simulink model "step6_ref"  (Simulink 10.2)
settings: Solver=FixedStepAuto  StartTime=0.0  StopTime=3  FixedStep=T_step  RelTol=1e-3
values from neighbouring files (symbols this model uses):
  gama0 = Rparams4dyn(3)    [PRBDM_3R_Dynamic_Matrices_Lagrange.m]    (also in PRBDM_3R_Dynamics.m = in4dyn(12); PRBDM_3R_Dynamics00.m = in4dyn(12); PRBDM_3R_DynamicsPID.m = in4dyn(12); PRBDM_3R_parameters.m = 0.1)
  gama1 = x(7)    [Jacobi_T.m]    (also in PRBDM_3R_Dynamic_Matrices_Lagrange.m = Rparams4dyn(4); PRBDM_3R_Dynamics.m = in4dyn(13); PRBDM_3R_Dynamics00.m = in4dyn(13); PRBDM_3R_DynamicsPID.m = in4dyn(13))
  gama2 = x(8)    [Jacobi_T.m]    (also in PRBDM_3R_Dynamic_Matrices_Lagrange.m = Rparams4dyn(5); PRBDM_3R_Dynamics.m = in4dyn(14); PRBDM_3R_Dynamics00.m = in4dyn(14); PRBDM_3R_DynamicsPID.m = in4dyn(14))
  gama3 = x(9)    [Jacobi_T.m]    (also in PRBDM_3R_Dynamic_Matrices_Lagrange.m = Rparams4dyn(6); PRBDM_3R_Dynamics.m = in4dyn(15); PRBDM_3R_Dynamics00.m = in4dyn(15); PRBDM_3R_DynamicsPID.m = in4dyn(15))
  I = Rparams4dyn(10)    [PRBDM_3R_Dynamic_Matrices_Lagrange.m]    (also in PRBDM_3R_Dynamics.m = in4dyn(19); PRBDM_3R_Dynamics00.m = in4dyn(19); PRBDM_3R_DynamicsPID.m = in4dyn(19); PRBDM_3R_parameters.m = 1.8e-11)
  k1 = Rparams4dyn(7)    [PRBDM_3R_Dynamic_Matrices_Lagrange.m]    (also in PRBDM_3R_Dynamics.m = in4dyn(16); PRBDM_3R_Dynamics00.m = in4dyn(16); PRBDM_3R_DynamicsPID.m = in4dyn(16); PRBDM_3R_parameters.m = 0.290628)
  k2 = Rparams4dyn(8)    [PRBDM_3R_Dynamic_Matrices_Lagrange.m]    (also in PRBDM_3R_Dynamics.m = in4dyn(17); PRBDM_3R_Dynamics00.m = in4dyn(17); PRBDM_3R_DynamicsPID.m = in4dyn(17); PRBDM_3R_parameters.m = 0.247572)
  k3 = Rparams4dyn(9)    [PRBDM_3R_Dynamic_Matrices_Lagrange.m]    (also in PRBDM_3R_Dynamics.m = in4dyn(18); PRBDM_3R_Dynamics00.m = in4dyn(18); PRBDM_3R_DynamicsPID.m = in4dyn(18); PRBDM_3R_parameters.m = 0.213624)
  L = Rparams4dyn(2)    [PRBDM_3R_Dynamic_Matrices_Lagrange.m]    (also in PRBDM_3R_Dynamics.m = in4dyn(11); PRBDM_3R_Dynamics00.m = in4dyn(11); PRBDM_3R_DynamicsPID.m = in4dyn(11); PRBDM_3R_parameters.m = 0.3)
  m = Rparams4dyn(1)    [PRBDM_3R_Dynamic_Matrices_Lagrange.m]    (also in PRBDM_3R_Dynamics.m = in4dyn(10); PRBDM_3R_Dynamics00.m = in4dyn(10); PRBDM_3R_DynamicsPID.m = in4dyn(10); PRBDM_3R_parameters.m = 1)
  W = x(22)    [PRBDM_3R_CTC.m]    (also in PRBDM_3R_Dynamic_Matrices_NewtonEular.m = robot_params(7); PRBDM_3R_Dynamics.m = in4dyn(20); PRBDM_3R_Dynamics00.m = in4dyn(20); PRBDM_3R_DynamicsPID.m = in4dyn(20))
libraries: pid_lib x1
settings Model: Creator=Master  LastModifiedBy=Master
settings DataIOCC: SaveFormat=Dataset  SignalLoggingSaveFormat=Dataset  ReturnWorkspaceOutputs=on
settings OptimizationCC: LifeSpan=auto
settings DebuggingCC: UnderspecifiedInitializationDetection=Simplified  MergeDetectMultiDrivingBlocksExec=error  FcnCallInpInsideContextMsg=error  SFUnexpectedBacktrackingDiag=error  SFNoUnconditionalDefaultTransitionDiag=error  SFExecutionAtInitializationDiag=warning  ArithmeticOperatorsInVariantConditions=error
settings HardwareCC: ProdBitPerPointer=64  ProdBitPerSizeT=64  ProdBitPerPtrDiffT=64  ProdLargestAtomicFloat=Float  ProdIntDivRoundTo=Zero  ProdEndianess=LittleEndian  ProdWordSize=64  ProdHWDeviceType=Intel->x86-64 (Windows64)
settings ModelReferenceCC: PropagateSignalLabelsOutOfModel=on
settings SFSimCC: SimUseLocalCustomCode=on  CustomCodeUndefinedFunction=FilterOut
settings RTWCC: RTWUseLocalCustomCode=on
settings CodeAppCC: StateflowObjectComments=off
settings GRTTargetCC: TargetLangStandard=C99 (ISO)  CombineOutputUpdateFcns=on  GRTInterface=off
settings ConfigComp: CovMetricSettings=dwe  CovSaveCumulativeToWorkspaceVar=off  CovSaveSingleToWorkspaceVar=off  CovExternalEMLEnable=on

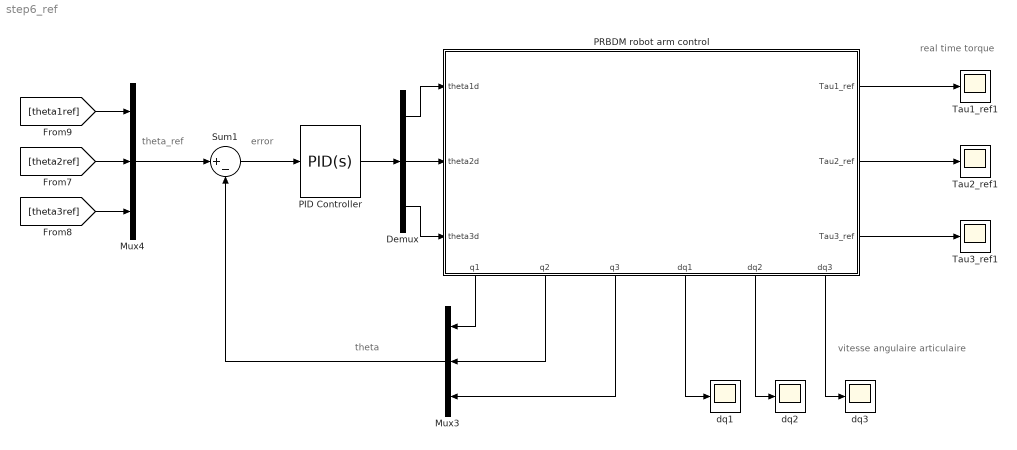
== system step6_ref ==
  note: vitesse angulaire articulaire
  note: real time torque
  note: theta
  note: theta_ref
  note: error
  " dq1" : Scope
  Demux : Demux  Outputs=3
  Mux3 : Mux  Inputs=3
  Mux4 : Mux  Inputs=3
  PID Controller : pid_lib/PID Controller  Controller=PID  Form=Parallel  TimeDomain=Continuous-time  UseExternalTs=off  SampleTime=-1  IntegratorMethod=Forward Euler  FilterMethod=Forward Euler  ControllerParametersSource=internal  P=1  I=1  D=0  UseFilter=on  N=100  TunerSelectOption=Transfer Function Based (PID Tuner App)  InitialConditionSource=internal  InitialConditionForIntegrator=0  InitialConditionForFilter=0  DifferentiatorICPrevScaledInput=0  ExternalReset=none  TrackingMode=off  Kt=1  LimitOutput=off  SatLimitsSource=internal  UpperSaturationLimit=inf  LowerSaturationLimit=-inf  LinearizeAsGain=on  AntiWindupMode=none  Kb=1  POutMin=[]  POutMax=[]  IOutMin=[]  IOutMax=[]  DOutMin=[]  DOutMax=[]  NOutMin=[]  NOutMax=[]  SumOutMin=[]  SumOutMax=[]  SaturationOutMin=[]  SaturationOutMax=[]  PParamMin=[]  PParamMax=[]  IParamMin=[]  IParamMax=[]  DParamMin=[]  DParamMax=[]  NParamMin=[]  NParamMax=[]  KbParamMin=[]  KbParamMax=[]  KtParamMin=[]  KtParamMax=[]  KbOutMin=[]  KbOutMax=[]  KtOutMin=[]  KtOutMax=[]  IntegratorOutMin=[]  IntegratorOutMax=[]  FilterOutMin=[]  FilterOutMax=[]  SumI1OutMin=[]  SumI1OutMax=[]  SumI2OutMin=[]  SumI2OutMax=[]  SumI3OutMin=[]  SumI3OutMax=[]  SumI4OutMin=[]  SumI4OutMax=[]  SumDOutMin=[]  SumDOutMax=[]  DifferentiatorOutMin=[]  DifferentiatorOutMax=[]  FilterDiffOutCoefMin=[]  FilterDiffOutCoefMax=[]  ReciprocalOutMin=[]  ReciprocalOutMax=[]  SumDenOutMin=[]  SumDenOutMax=[]  SumNumOutMin=[]  SumNumOutMax=[]  DivideOutMin=[]  DivideOutMax=[]  UdiffTsProdOutMin=[]  UdiffTsProdOutMax=[]  NTsProdOutMin=[]  NTsProdOutMax=[]  UintegralTsProdOutMin=[]  UintegralTsProdOutMax=[]  UngainTsProdOutMin=[]  UngainTsProdOutMax=[]  IntegratorContinuousStateAttributes=''  IntegratorStateMustResolveToSignalObject=off  IntegratorRTWStateStorageClass=Auto  FilterContinuousStateAttributes=''  FilterStateMustResolveToSignalObject=off  FilterRTWStateStorageClass=Auto  ParallelPVariant=InternalParameters  IdealPVariant=Disabled  IVariant=InternalParameters  DVariant=InternalParameters  IntegratorVariant=Continuous  SatVariant=Disabled  AWVariant=Passthrough  PCopyVariant=Disabled  TRVariant=Disabled  FdbkBlocksVariant=Forward  IdealPFdbkVariant=Disabled  SatFdbkVariant=Disabled  DerivativeFilterVariant=ContFilter  NVariant=InternalParameters  NCopyVariant=Disabled  FilterICVariant=InternalICsFilter  IntegratorICVariant=InternalICs  ExternalResetVariant=Disabled  TRSumVariant=Passthrough  SumFdbkVariant=Disabled  SumVariant=Sum_PID  TsampFilterVariant=InternalTs  TsampNgainVariant=Passthrough  TsampIntegralVariant=Passthrough  ExternalSaturationOutDataTypeStr=Inherit: Same as second input
  PRBDM robot arm control : Subsystem
      settings: PortSchema="{\"entries\":[{\"content\":{\"sides\":[{\"content\":{\"connectorIds\":[\"In1\",\"In2\",\"In3\"]},\"type\":\"ConnectorPlacement.EquallySpacedRectSide\",\"uuid\":\"1e89617d-77c4-4021-ad02-b23032c49c13\"},{\"content\":{\"connectorIds\":[\"Out1\",\"Out2\",\"Out3\"],\"side\":\"RIGHT\"},\"type\":\"ConnectorPlacement.EquallySpacedRectSide\",\"uuid\":\"af1c966f-61d8-4dd1-b14e-ca4c94ca536d\"},{\"content\":{\"connectorIds\":[],\"side\":\"TOP\"},\"type\":\"ConnectorPlacement.EquallySpacedRectSide\",\"uuid\":\"dae36e8b-a61f-4fb2-b828-973ce72430cd\"},{\"content\":{\"connectorIds\":[\"Out4\",\"Out5\",\"Out6\",\"Out7\",\"Out8\",\"Out9\"],\"side\":\"BOTTOM\"},\"type\":\"ConnectorPlacement.EquallySpacedRectSide\",\"uuid\":\"432115d0-4cd6-420b-9ede-52c2ebd6cc12\"},{\"content\":{\"connectorIds\":[],\"side\":\"HIDDEN\"},\"type\":\"ConnectorPlacement.EquallySpacedRectSide\",\"uuid\":\"bc2aa4ed-b8ff-4e0b-a675-9c9f1376083d\"}]},\"type\":\"ConnectorPlacement.EquallySpacedConnector\",\"uuid\":\"b45c6bc8-8dc8-4362-beb6-c8f75c6afe37\"}],\"packageUris\":[\"http://schema.mathworks.com/mf0/Connector/R2020b\"],\"version\":\"1.0\"}"
      mask Display: image(imread('RRR.png'))
  Sum1 : Sum  Inputs=|+-
  Tau1_ref1 : Scope
  Tau2_ref1 : Scope
  Tau3_ref1 : Scope
  dq2 : Scope
  dq3 : Scope
  wires:
  PRBDM robot arm control/4(q1) -> Mux3/1
  [theta2ref] -> Mux4/2
  [theta3ref] -> Mux4/3
  [theta1ref] -> Mux4/1
  Mux4/1 -> Sum1/1
  Mux3/1 -> Sum1/2
  Sum1/1 -> PID Controller/1
  PID Controller/1 -> Demux/1
  Demux/2 -> PRBDM robot arm control/2(theta2d)
  Demux/1 -> PRBDM robot arm control/1(theta1d)
  Demux/3 -> PRBDM robot arm control/3(theta3d)
  PRBDM robot arm control/5(q2) -> Mux3/2
  PRBDM robot arm control/6(q3) -> Mux3/3
  PRBDM robot arm control/7(dq1) -> " dq1"/1
  PRBDM robot arm control/8(dq2) -> dq2/1
  PRBDM robot arm control/9(dq3) -> dq3/1
  PRBDM robot arm control/2(Tau2_ref) -> Tau2_ref1/1
  PRBDM robot arm control/1(Tau1_ref) -> Tau1_ref1/1
  PRBDM robot arm control/3(Tau3_ref) -> Tau3_ref1/1

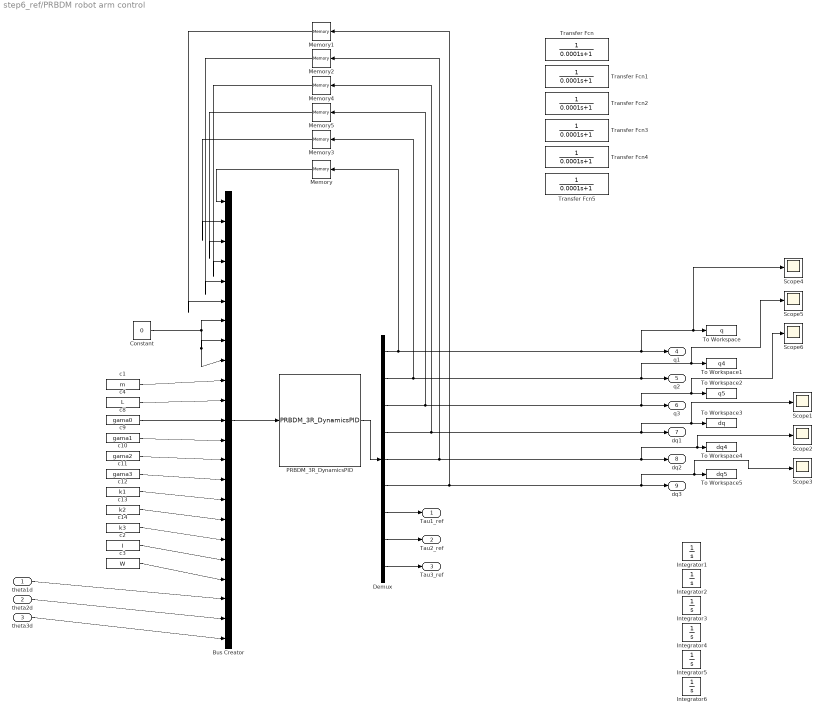
== system step6_ref/PRBDM robot arm control ==
  theta1d : Inport
  theta2d : Inport  Port=2
  theta3d : Inport  Port=3
  Bus Creator : BusCreator  Inputs=23
  Constant : Constant  Value=0
  Demux : Demux  Outputs=9
  Integrator{1..6} (6 alike) : Integrator  UpperSaturationLimit=1e6  LowerSaturationLimit=-1e6
  Memory{,1..5} (6 alike) : Memory
  PRBDM_3R_DynamicsPID : MATLABFcn  MATLABFcn=PRBDM_3R_DynamicsPID  OutputDimensions=9
  Scope{1..6} (6 alike) : Scope
  To Workspace : ToWorkspace  VariableName=q  SampleTime=-1
  To Workspace1 : ToWorkspace  VariableName=q4  SampleTime=-1
  To Workspace2 : ToWorkspace  VariableName=q5  SampleTime=-1
  To Workspace3 : ToWorkspace  VariableName=dq  SampleTime=-1
  To Workspace4 : ToWorkspace  VariableName=dq4  SampleTime=-1
  To Workspace5 : ToWorkspace  VariableName=dq5  SampleTime=-1
  Transfer Fcn{,1..5} (6 alike) : TransferFcn  Denominator=[0.0001 1]
  c1 : Constant  Value=m
  c10 : Constant  Value=gama2
  c11 : Constant  Value=gama3
  c12 : Constant  Value=k1
  c13 : Constant  Value=k2
  c14 : Constant  Value=k3
  c2 : Constant  Value=I
  c3 : Constant  Value=W
  c4 : Constant  Value=L
  c8 : Constant  Value=gama0
  c9 : Constant  Value=gama1
  Tau1_ref : Outport
  Tau2_ref : Outport  Port=2
  Tau3_ref : Outport  Port=3
  q1 : Outport  Port=4
  q2 : Outport  Port=5
  q3 : Outport  Port=6
  dq1 : Outport  Port=7
  dq2 : Outport  Port=8
  dq3 : Outport  Port=9
  wires:
  theta3d/1 -> Bus Creator/23
  theta2d/1 -> Bus Creator/22
  c11/1 -> Bus Creator/15
  c3/1 -> Bus Creator/20
  c14/1 -> Bus Creator/18
  c2/1 -> Bus Creator/19
  c1/1 -> Bus Creator/10
  c8/1 -> Bus Creator/12
  Bus Creator/1 -> PRBDM_3R_DynamicsPID/1
  PRBDM_3R_DynamicsPID/1 -> Demux/1
  c4/1 -> Bus Creator/11
  c10/1 -> Bus Creator/14
  c9/1 -> Bus Creator/13
  c13/1 -> Bus Creator/17
  c12/1 -> Bus Creator/16
  theta1d/1 -> Bus Creator/21
  Demux/1 -> Memory/1, q1/1, Scope4/1, To Workspace/1
  Demux/2 -> Memory3/1, q2/1, Scope5/1, To Workspace1/1
  Demux/3 -> Memory5/1, q3/1, Scope6/1, To Workspace2/1
  Demux/4 -> Memory4/1, dq1/1, Scope1/1, To Workspace3/1
  Demux/5 -> Memory2/1, dq2/1, Scope2/1, To Workspace4/1
  Demux/6 -> Memory1/1, dq3/1, Scope3/1, To Workspace5/1
  Memory/1 -> Bus Creator/1
  Memory3/1 -> Bus Creator/2
  Memory5/1 -> Bus Creator/3
  Memory4/1 -> Bus Creator/4
  Memory2/1 -> Bus Creator/5
  Memory1/1 -> Bus Creator/6
  Demux/7 -> Tau1_ref/1
  Demux/8 -> Tau2_ref/1
  Demux/9 -> Tau3_ref/1
  Constant/1 -> Bus Creator/9, Bus Creator/8, Bus Creator/7
